simulink model "Closed_Loop_TF_Noise"  (R2023a)
settings: Solver=VariableStepAuto  StartTime=0.0  StopTime=10.0  RelTol=1e-3
undefined symbols (not defined in the file): a, b, d, K, M
settings Model: Creator=m260477  LastModifiedBy=m260477

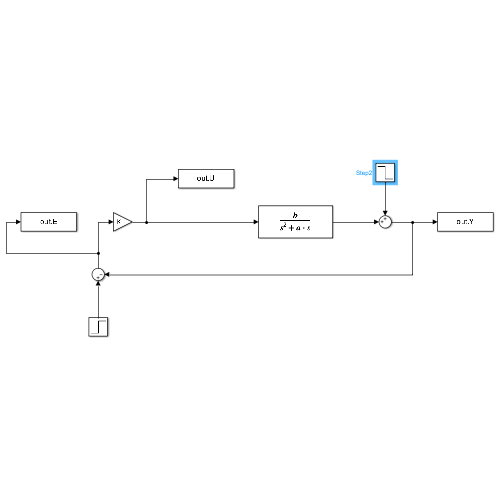
[thumbnail: Simulink's stored preview of the top-level diagram]
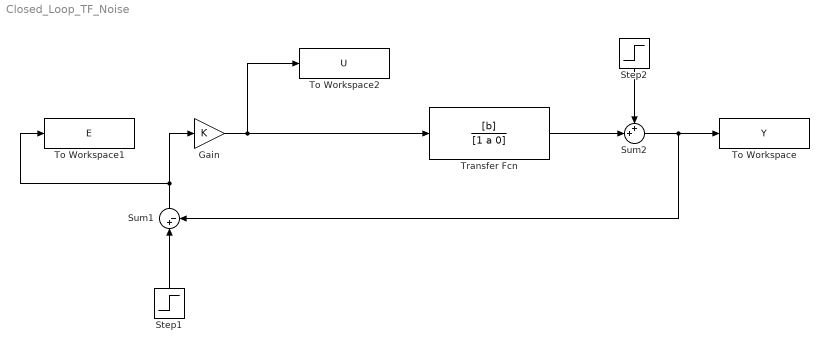
== system Closed_Loop_TF_Noise ==
  Gain : Gain  Gain=K
  Step1 : Step  Time=0  After=M  SampleTime=0
  Step2 : Step  Time=0  After=d  SampleTime=0
  Sum1 : Sum  Inputs=|+-
  Sum2 : Sum  Inputs=++|
  To Workspace : ToWorkspace  VariableName=Y  SaveFormat=Timeseries  SampleTime=-1
  To Workspace1 : ToWorkspace  VariableName=E  SaveFormat=Timeseries  SampleTime=-1
  To Workspace2 : ToWorkspace  VariableName=U  SaveFormat=Timeseries  SampleTime=-1
  Transfer Fcn : TransferFcn  Numerator=[b]  Denominator=[1 a 0]
  wires:
  Step1/1 -> Sum1/1
  Gain/1 -> Transfer Fcn/1, To Workspace2/1
  Sum1/1 -> To Workspace1/1, Gain/1
  Sum2/1 -> Sum1/2, To Workspace/1
  Transfer Fcn/1 -> Sum2/2
  Step2/1 -> Sum2/1
